simulink model "MultirotorModel"  (R2022b)
settings: Solver=VariableStepAuto  StartTime=0.0  StopTime=200  FixedStep=0.005  RelTol=1e-3  EnableMultiTasking=on
undefined symbols (not defined in the file): Controller, decyear, DiscIntNeverNeededParam, DroneMass, Dz, Earth, Gravity, initialConditions, Iz, leapyear, Nz, Pz, startFlightTime, UAVSampleTime, Vehicle, WGS84
libraries: slpidlib x10, uavalgslib x7, simulink x2, sharedutil x2, aerolibconvert2 x2, aerolibtransform2 x2, aerolibatmos2 x1, aerolibgravity2 x1, shared6dof x1, aerolibasang x1, sensorinslib x1
(part 3 of 3)

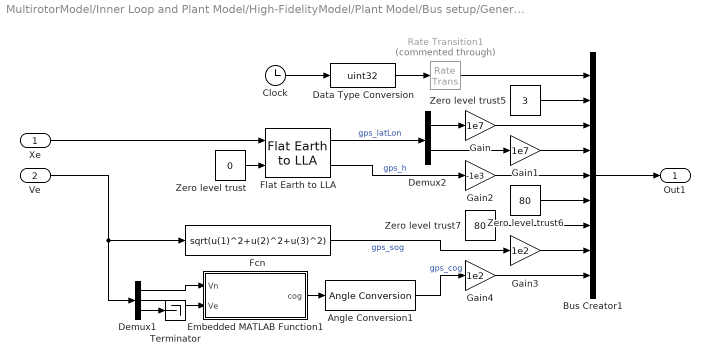
== system MultirotorModel/Inner Loop and Plant Model/High-FidelityModel/Plant Model/Bus setup/Generate GPS Data/Scale and Assemble GPS Data  ==
  Xe : Inport
  Ve : Inport  Port=2
  Angle Conversion1 : aerolibconvert2/Angle Conversion  IU=rad  OU=deg
  Bus Creator1 : BusCreator  Inputs=9  OutDataTypeStr=Bus: gps_raw_int  NonVirtualBus=on
      settings: InheritFromInputs=off
  Clock : Clock
      settings: AttributesFormatString=Decimation: %<Decimation>
  Data Type Conversion : DataTypeConversion  OutDataTypeStr=uint32  SaturateOnIntegerOverflow=off  RndMeth=Floor
  Demux1 : Demux  Outputs=3
  Demux2 : Demux  Outputs=2
  Embedded MATLAB Function1 : MATLAB Function  TreatAsAtomicUnit=on
  Fcn : Fcn  Expr=sqrt(u(1)^2+u(2)^2+u(3)^2)
  Flat Earth to LLA : aerolibtransform2/Flat Earth to LLA  units=Metric (MKS)  ptype=Earth (WGS84)  F=1/298.257223563  R=6378137  refPosPort=off  LL0=uavIC_latLon  psi=0
  Gain : Gain  Gain=1e7  OutDataTypeStr=int32
  Gain1 : Gain  Gain=1e7  OutDataTypeStr=int32
  Gain2 : Gain  Gain=-1e3  OutDataTypeStr=int32
  Gain3 : Gain  Gain=1e2  OutDataTypeStr=uint16
  Gain4 : Gain  Gain=1e2  OutDataTypeStr=uint16
  Rate Transition1 : RateTransition  Commented=through  OutPortSampleTime=0.005
  Terminator : Terminator
  Zero level trust : Constant  Value=0
      settings: AttributesFormatString=%<Value>
  Zero level trust5 : Constant  Value=3  OutDataTypeStr=uint8
      settings: AttributesFormatString=%<Value>
  Zero level trust6 : Constant  Value=80  OutDataTypeStr=uint16
      settings: AttributesFormatString=%<Value>
  Zero level trust7 : Constant  Value=80  OutDataTypeStr=uint16
      settings: AttributesFormatString=%<Value>
  Out1 : Outport
  wires:
  Demux2/1 -> Gain/1
  Gain/1 -> Bus Creator1/3
  Gain4/1 -> Bus Creator1/9
  Demux2/2 -> Gain1/1
  Embedded MATLAB Function1/1(cog) -> Angle Conversion1/1
  Rate Transition1/1 -> Bus Creator1/1
  Zero level trust6/1 -> Bus Creator1/6
  Gain3/1 -> Bus Creator1/8
  Clock/1 -> Data Type Conversion/1
  Ve/1 -> Demux1/1, Fcn/1
  Zero level trust7/1 -> Bus Creator1/7
  Data Type Conversion/1 -> Rate Transition1/1
  Demux1/2 -> Embedded MATLAB Function1/2(Ve)
  Zero level trust5/1 -> Bus Creator1/2
  Demux1/1 -> Embedded MATLAB Function1/1(Vn)
  Flat Earth to LLA/1 -> Demux2/1  "gps_latLon"
  Gain2/1 -> Bus Creator1/5
  Fcn/1 -> Gain3/1  "gps_sog"
  Gain1/1 -> Bus Creator1/4
  Flat Earth to LLA/2 -> Gain2/1  "gps_h"
  Zero level trust/1 -> Flat Earth to LLA/2
  Angle Conversion1/1 -> Gain4/1  "gps_cog"
  Demux1/3 -> Terminator/1
  Xe/1 -> Flat Earth to LLA/1
  Bus Creator1/1 -> Out1/1

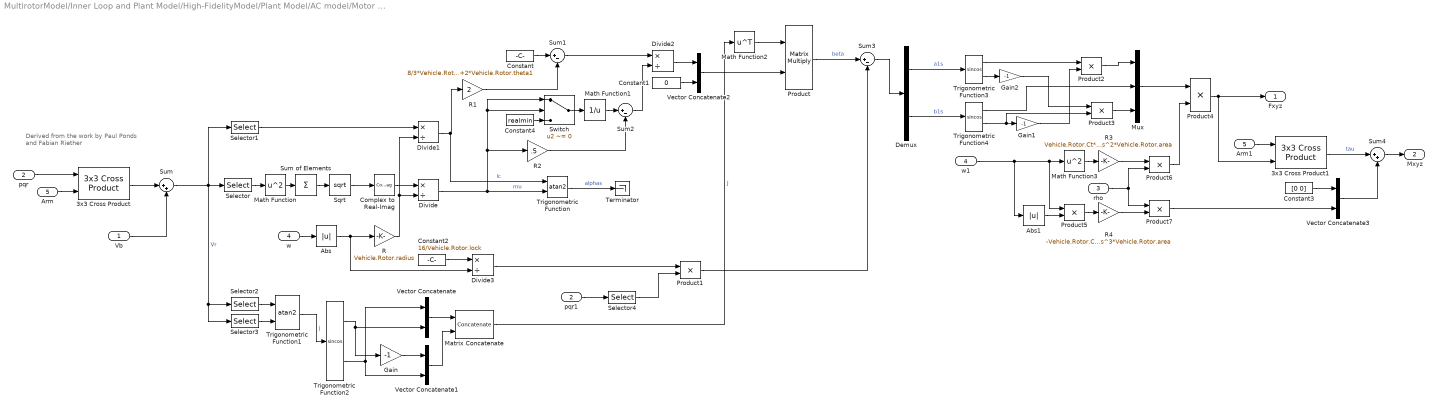
== system MultirotorModel/Inner Loop and Plant Model/High-FidelityModel/Plant Model/AC model/Motor Forces and Torques/For Each Subsystem/RotorDynamics ==
  note: Derived from the work by Paul Ponds
      | and Fabian Riether
  Vb : Inport  PortDimensions=3
  pqr : Inport  Port=2  PortDimensions=3
  rho : Inport  Port=3  PortDimensions=1
  w : Inport  Port=4  PortDimensions=[1 1]
  Arm : Inport  Port=5  PortDimensions=[3 1]
  3x3 Cross Product : sharedutil/3x3 Cross Product  aMode=aMode
  3x3 Cross Product1 : sharedutil/3x3 Cross Product  aMode=aMode
  Abs : Abs  SaturateOnIntegerOverflow=off
  Abs1 : Abs  SaturateOnIntegerOverflow=off
  Arm1 : InportShadow  Port=5  PortDimensions=[3 1]
  Complex to Real-Imag : ComplexToRealImag  Output=Real
  Constant : Constant  Value=8/3*Vehicle.Rotor.theta0+2*Vehicle.Rotor.theta1
  Constant1 : Constant  Value=0
  Constant2 : Constant  Value=16/Vehicle.Rotor.lock
  Constant3 : Constant  Value=[0 0]
  Constant4 : Constant  Value=realmin
  Demux : Demux  Outputs=2
  Divide{,1..3} (4 alike) : Product  Inputs=*/
  Gain : Gain  Gain=-1
  Gain1 : Gain  Gain=-1
  Gain2 : Gain  Gain=-1
  Math Function : Math  Operator=square  SignedPower=on
  Math Function1 : Math  Operator=reciprocal  SignedPower=on
  Math Function2 : Math  Operator=transpose  SignedPower=on
  Math Function3 : Math  Operator=square  SignedPower=on
  Matrix Concatenate : Concatenate  Mode=Multidimensional array  ConcatenateDimension=2
  Mux : Mux  Inputs=3
  Product : Product  Multiplication=Matrix(*)
  Product{1..7} (7 alike) : Product
  R : Gain  Gain=Vehicle.Rotor.radius
  R1 : Gain  Gain=2
  R2 : Gain  Gain=.5
  R3 : Gain  Gain=Vehicle.Rotor.Ct*Vehicle.Rotor.radius^2*Vehicle.Rotor.area
  R4 : Gain  Gain=-Vehicle.Rotor.Cq*Vehicle.Rotor.radius^3*Vehicle.Rotor.area
  Selector : Selector  InputPortWidth=3  IndexOptions=Index vector (dialog)  Indices=[1 2]  OutputSizes=1
  Selector1 : Selector  InputPortWidth=3  IndexOptions=Index vector (dialog)  Indices=[3]  OutputSizes=1
  Selector2 : Selector  InputPortWidth=3  IndexOptions=Index vector (dialog)  Indices=[2]  OutputSizes=1
  Selector3 : Selector  InputPortWidth=3  IndexOptions=Index vector (dialog)  Indices=[1]  OutputSizes=1
  Selector4 : Selector  InputPortWidth=3  IndexOptions=Index vector (dialog)  Indices=[2 1]  OutputSizes=1
  Sqrt : Sqrt  OutputSignalType=complex
  Sum : Sum  Inputs=|++
  Sum of Elements : Sum  Inputs=+
  Sum1 : Sum  Inputs=|+-
  Sum2 : Sum  Inputs=|+-
  Sum3 : Sum  Inputs=|+-
  Sum4 : Sum  Inputs=|++
  Switch : Switch  Criteria=u2 ~= 0  SaturateOnIntegerOverflow=off  InputSameDT=off
  Terminator : Terminator
  Trigonometric Function : Trigonometry  Operator=atan2
  Trigonometric Function1 : Trigonometry  Operator=atan2
  Trigonometric Function2 : Trigonometry  Operator=sincos
  Trigonometric Function3 : Trigonometry  Operator=sincos
  Trigonometric Function4 : Trigonometry  Operator=sincos
  Vector Concatenate{,1..3} (4 alike) : Concatenate
  pqr1 : InportShadow  Port=2  PortDimensions=3
  w1 : InportShadow  Port=4  PortDimensions=[1 1]
  Fxyz : Outport  PortDimensions=[3 1]  VectorParamsAs1DForOutWhenUnconnected=off
  Mxyz : Outport  Port=2  PortDimensions=[3 1]  VectorParamsAs1DForOutWhenUnconnected=off
  wires:
  Complex to Real-Imag/1 -> Divide/1
  Sqrt/1 -> Complex to Real-Imag/1
  Constant4/1 -> Switch/3
  Switch/1 -> Math Function1/1
  Product1/1 -> Sum3/2
  rho/1 -> Product7/1, Product6/2
  Product7/1 -> Vector Concatenate3/2
  Product6/1 -> Product4/2
  Sum4/1 -> Mxyz/1
  3x3 Cross Product1/1 -> Sum4/1  "tau"
  Product4/1 -> Fxyz/1, 3x3 Cross Product1/2
  Arm1/1 -> 3x3 Cross Product1/1
  Vector Concatenate3/1 -> Sum4/2
  Constant3/1 -> Vector Concatenate3/1
  R4/1 -> Product7/2
  Product5/1 -> R4/1
  Abs1/1 -> Product5/2
  R3/1 -> Product6/1
  Mux/1 -> Product4/1
  Gain2/1 -> Product3/1
  Product3/1 -> Mux/3
  Trigonometric Function3/2 -> Gain2/1
  Trigonometric Function4/1 -> Mux/2
  Product2/1 -> Mux/1
  Trigonometric Function3/1 -> Product2/1
  Gain1/1 -> Product2/2
  Trigonometric Function4/2 -> Gain1/1, Product3/2
  Demux/2 -> Trigonometric Function4/1  "b1s"
  Demux/1 -> Trigonometric Function3/1  "a1s"
  Sum3/1 -> Demux/1
  Math Function3/1 -> R3/1
  w1/1 -> Math Function3/1, Product5/1, Abs1/1
  Divide3/1 -> Product1/1
  Abs/1 -> R/1, Divide3/2
  Selector4/1 -> Product1/2
  pqr1/1 -> Selector4/1
  Constant2/1 -> Divide3/1
  Product/1 -> Sum3/1  "beta"
  Math Function2/1 -> Product/1
  Vector Concatenate2/1 -> Product/2
  Constant1/1 -> Vector Concatenate2/2
  Divide2/1 -> Vector Concatenate2/1
  Sum2/1 -> Divide2/2
  R2/1 -> Sum2/2
  Math Function1/1 -> Sum2/1
  Sum1/1 -> Divide2/1
  R1/1 -> Sum1/2
  Constant/1 -> Sum1/1
  Matrix Concatenate/1 -> Math Function2/1  "J"
  Vector Concatenate1/1 -> Matrix Concatenate/2
  Vector Concatenate/1 -> Matrix Concatenate/1
  Trigonometric Function2/1 -> Gain/1, Vector Concatenate/2
  Gain/1 -> Vector Concatenate1/1
  Trigonometric Function2/2 -> Vector Concatenate/1, Vector Concatenate1/2
  Trigonometric Function1/1 -> Trigonometric Function2/1  "j"
  Selector3/1 -> Trigonometric Function1/2
  Selector2/1 -> Trigonometric Function1/1
  Trigonometric Function/1 -> Terminator/1  "alphas"
  Divide1/1 -> Trigonometric Function/1, R1/1  "lc"
  Selector1/1 -> Divide1/1
  Divide/1 -> Trigonometric Function/2, Switch/1, Switch/2, R2/1  "mu"
  R/1 -> Divide/2, Divide1/2
  w/1 -> Abs/1
  Arm/1 -> 3x3 Cross Product/2
  pqr/1 -> 3x3 Cross Product/1
  Sum of Elements/1 -> Sqrt/1
  Math Function/1 -> Sum of Elements/1
  Selector/1 -> Math Function/1
  Sum/1 -> Selector/1, Selector1/1, Selector2/1, Selector3/1  "Vr"
  Vb/1 -> Sum/2
  3x3 Cross Product/1 -> Sum/1

== matlab function MultirotorModel/Guidance Logic/Full Guidance Logic/Guidance Stateflow/Guidance Mode Selector/GuidanceLogic.Land.ToLand/MATLAB Function ==
  data: FromWP input Bus: uavPathManagerBus size=1; wps output; ToWP input Bus: uavPathManagerBus size=1
function wps = getLandingWaypoint(FromWP, ToWP)

persistent outWPS

if isempty(outWPS)
    outWPS = single(zeros(2,4));
end

outWPS(1,:) = [FromWP.position' FromWP.params(4)];
outWPS(2,:) = [ToWP.position(1:2)' FromWP.position(3) ToWP.params(4)];

wps = outWPS;

== matlab function MultirotorModel/Guidance Logic/Full Guidance Logic/Guidance Stateflow/Guidance Mode Selector/GuidanceLogic.WP/MATLAB Function ==
  data: FromWP input Bus: uavPathManagerBus size=1; wps output; ToWP input Bus: uavPathManagerBus size=1
function wps = getWaypointMission(FromWP, ToWP)

persistent outWPS

if isempty(outWPS)
    outWPS = single(zeros(2,4));
end

outWPS(1,:) = [FromWP.position' FromWP.params(4)];
outWPS(2,:) = [ToWP.position' ToWP.params(4)];

% for ii=1:2
%     outWPS(ii,1:3) = GCSMission(ii).position';
%     outWPS(ii,4) = GCSMission(ii).params(4);
% end

wps = outWPS;

== matlab function MultirotorModel/Guidance Logic/Obstacle Avoidance3D/MATLAB Function ==
  data: mission input; Steer input size=[5 1]; y output; UAVState input; DTD output; needHover output
function [y, DTD, needHover] = computeLPWaypoints(mission, Steer,UAVState)
%#codegen

Wp1 = [mission(1).position' mission(1).params(4)];
Wp2x = mission(2).position(1);
Wp2y = mission(2).position(2);
needHover = false;

% Follow obstacle avoidance steer direction when UAV is above 5 meters
% above ground
if (~any(isnan(Steer)) && (UAVState.z < -5))
    if (Steer(5) == 0)
        % Compute look ahead point 6 meters along the steering direction
        LAP_local = 6*Steer(2:4)';
        % Follow yaw command from obstacle avoidance
        yaw = Steer(1);
        LAP = [LAP_local yaw] + [UAVState.x, UAVState.y, UAVState.z, 0];
        if(isnan(LAP(4)))
            LAP(4) = 0;
        end

        y = [ Wp1(1,:) ; LAP ; Wp2x , Wp2y , 0 , LAP(4) ];
        DTD = norm([Wp2x Wp2y] - LAP(1:2));
    else
        % Rotate in place
        y = [ Wp1(1,:) ; UAVState.x, UAVState.y, UAVState.z Steer(1); Wp2x , Wp2y , 0 , Steer(1) ];
        DTD = norm([Wp2x Wp2y] - [UAVState.x, UAVState.y]);
        needHover = true;
    end
    
else
    % If there is no good steer direction or UAV is too low, fly up
    y = [ Wp1(1,:) ; UAVState.x , UAVState.y , UAVState.z-2 , 0 ; Wp2x , Wp2y , 0 , 0 ];
    DTD = norm([Wp2x Wp2y] - [UAVState.x, UAVState.y]);
end

if(DTD<5)
    % When close to target point, switch to landing
    y = [ Wp1(1,:) ; Wp2x , Wp2y, -11 , 0 ; Wp2x , Wp2y , -1 , 0 ];
end


end

== matlab function MultirotorModel/Inner Loop and Plant Model/Low-FidelityModel/Assemble UAV State Bus/Generate GPS Data/Embedded MATLAB Function1 ==
  data: cog output; Vn input; Ve input
function cog = getCOG(Vn, Ve)
% This block supports an embeddable subset of the MATLAB language.
% See the help menu for details. 

cog = atan2(Ve,Vn);
if cog < 0;
    cog = cog + 2*pi;
end

== matlab function MultirotorModel/Guidance Logic/Obstacle Avoidance/MATLAB Function ==
  data: mission input; Steer input; y output; UAVState input
function y = computeLPWaypoints(mission, Steer,UAVState)
%#codegen

Wp1 = [mission(1).position' mission(1).params(4)];
Wp2x = mission(2).position(1);
Wp2y = mission(2).position(2);

if(~isnan(Steer))
    
    LAP_local = 6*[cos(Steer), sin(Steer)];
    LAP = [ LAP_local(1)+ UAVState.x , LAP_local(2) + UAVState.y , -11 , Steer];   
    if(isnan(LAP(4)))
        LAP(4) = 0;
    end
   
    y = [ Wp1(1,:) ; LAP ; Wp2x , Wp2y , 0 , Steer ];    
    DTD = sqrt( (LAP(1) - Wp2x)^2 + (LAP(2)-Wp2y)^2);  
    
else
    y = [ Wp1(1,:) ; UAVState.x , UAVState.y , UAVState.z-2 , 0 ; Wp2x , Wp2y , 0 , 0 ];
    DTD = sqrt( (UAVState.x - Wp2x)^2 + (UAVState.y-Wp2y)^2);
end

if(DTD<5)
    y = [ Wp1(1,:) ; Wp2x , Wp2y, -11 , 0 ; Wp2x , Wp2y , 0 , 0 ];
end


end

== matlab function MultirotorModel/Inner Loop and Plant Model/Low-FidelityModel/Position and Acceleration Control/Attitude Control/Multirotor Acceleration Control ==
  data: acc input; roll output; pitch output; yaw input; Gravity parameter
function [roll, pitch] = accControl(acc, yaw, Gravity)

    xddot = acc(1);
    yddot = acc(2);
    zddot = acc(3);
    
    pitch = atan2((-xddot*cos(yaw)-yddot*sin(yaw)), ( -zddot + Gravity));
    roll = atan2(((-xddot*sin(yaw)+yddot*cos(yaw))*cos(pitch)), (-zddot+Gravity));
    
end

== matlab function MultirotorModel/Inner Loop and Plant Model/Low-FidelityModel/Position and Acceleration Control/Attitude Control/Multirotor Thrust Control ==
  data: acc input; pitch input; thrust output; roll input; DroneMass parameter; Gravity parameter
function thrust  = thrustControl(acc, pitch, roll, DroneMass, Gravity)

    zddot = acc(3);
    
    thrust = DroneMass*(-zddot+Gravity)/(cos(pitch)*cos(roll));
end

== matlab function MultirotorModel/Inner Loop and Plant Model/High-FidelityModel/Control System/Controller/Position Controller/Position error transformation (Earth to Body frame) ==
  data: yaw input; xy_err_earth input; xy_err_body output
function xy_err_body = LTP2B2D(yaw,xy_err_earth)

transformation = [cos(yaw), sin(yaw); -sin(yaw),  cos(yaw)];
xy_err_body = transformation * xy_err_earth;


end

== matlab function MultirotorModel/Inner Loop and Plant Model/High-FidelityModel/Control System/Controller/Position Controller/Velocity error transformation (Earth to Body frame) ==
  data: yaw input; xy_err_earth input; xy_err_body output
function xy_err_body = LTP2B2D(yaw,xy_err_earth)

transformation = [cos(yaw), sin(yaw); -sin(yaw),  cos(yaw)];
xy_err_body = transformation * xy_err_earth;


end

== matlab function MultirotorModel/Inner Loop and Plant Model/High-FidelityModel/Control System/Controller/Yaw Controller/MATLAB Function ==
  data: u input; y output
function y = wrapYaw(u)
%u error in rad in -2pi to 2pi

if (u>pi)
    y = u-2*pi;
elseif(u<-pi)
    y = u +2*pi;
else
    y=u;
end

== matlab function MultirotorModel/Inner Loop and Plant Model/High-FidelityModel/Control System/Controller/Yaw Controller/MATLAB Function1 ==
  data: u input; y output
function y = wrapYaw(u)
%u error in rad in -2pi to 2pi

if (u>pi)
    y = u-2*pi;
elseif(u<-pi)
    y = u +2*pi;
else
    y=u;
end

== matlab function MultirotorModel/Inner Loop and Plant Model/High-FidelityModel/Plant Model/Bus setup/Generate GPS Data/Scale and Assemble GPS Data /Embedded MATLAB Function1 ==
  data: cog output; Vn input; Ve input
function cog = getCOG(Vn, Ve)
% This block supports an embeddable subset of the MATLAB language.
% See the help menu for details. 

cog = atan2(Ve,Vn);
if cog < 0;
    cog = cog + 2*pi;
end

== stateflow chart MultirotorModel/Guidance Logic/Full Guidance Logic/Guidance Stateflow/Guidance Mode Selector ==
  settings: updateMethod=DISCRETE  sampleTime=UAVSampleTime*4
  state GuidanceLogic
    state OnGround
    state Takeoff
    state WP
    state Orbit
    state Land
      state ToLand
      state Descend
      (default) -> ToLand
      ToLand -> Descend : [norm(Pose(1:2)-ToWP.position(1:2)) <= 5]
    (default) -> OnGround
    OnGround -> (junction 5) : [startFlight==1]
    Takeoff -> WP : [Pose(3) <= ToWP.position(3)]{Status = 1;}
    GuidanceLogic -> (junction 5) : [hasChanged(mode)]
    (junction 5) -> Takeoff [order 1] : [mode == 1]
    (junction 5) -> (junction 12) [order 2]
    (junction 12) -> WP [order 1] : [mode==2]
    (junction 12) -> (junction 17) [order 2]
    (junction 17) -> Orbit [order 1] : [mode==3]
    (junction 17) -> (junction 22) [order 2]
    (junction 22) -> Land
    Land -> GuidanceLogic : [Pose(3)>=-0.1]{Status = 2;}
  (default) -> GuidanceLogic
  data: sf_internal_action_state_placeholder_data local double size=1 =0; sf_internal_action_state_placeholder_data local double size=1 =0; sf_internal_action_state_placeholder_data local double size=1 =0; sf_internal_action_state_placeholder_data local double size=1 =0; sf_internal_action_state_placeholder_data local double size=1 =0; mode input; ToWP input Bus: uavPathManagerBus; InnerLoopCmds output Bus: innerLoopCmdsBus; Status output uint8; FromWP input Bus: uavPathManagerBus; Pose input; startFlight input; GdncMode output Enum: GdncModeType
